simulink model "sgMdl_IO750_EtherCATDriveControl"  (R2024b)
settings: Solver=FixedStepAuto  StartTime=0.0  StopTime=inf  RelTol=1e-3  EnableMultiTasking=on
undefined symbols (not defined in the file): AUS0, AUS1, C, DiscIntNeverNeededParam, padding, sigbuilder_block, Statuswort, Steuerwort, Ts
libraries: slrealtimeethercatlib x13, simulink x10, speedgoatlib_IO750 x5, speedgoatlib_shared x1
Description:
  | IO750 - EtherCAT Drive Control
settings Model: ModifiedByFormat=Speedgoat  SimulationMode=external  Creator=Speedgoat  LastModifiedBy=Speedgoat
settings SolverCC: ConcurrentTasks=on  AlgebraicLoopSolver=TrustRegion  PositivePriorityOrder=on  AutoInsertRateTranBlk=on
settings DataIOCC: SaveFormat=StructureWithTime
settings OptimizationCC: BlockReduction=off  OptimizeBlockIOStorage=off  BufferReuse=off  GlobalBufferReuse=off  ExpressionFolding=off  LocalBlockOutputs=off  OptimizeDataStoreBuffers=off  BusAssignmentInplaceUpdate=off
settings DebuggingCC: TasksWithSamePriorityMsg=none  UnconnectedInputMsg=warning  UnconnectedOutputMsg=warning  UnconnectedLineMsg=warning
settings HardwareCC: ProdBitPerLong=64  ProdLongLongMode=on  ProdHWDeviceType=Intel->x86-64 (Linux 64)
settings ModelReferenceCC: EnableRefExpFcnMdlSchedulingChecks=on
settings RTWCC: Description=Speedgoat Real-Time Target Machine  SystemTargetFile=speedgoat.tlc  TemplateMakefile=slrealtime_default_tmf  Toolchain=Simulink Real-Time Toolchain  BuildConfiguration=Faster Runs  TargetLang=C++  GPUComputeCapability=3.5  DLArmComputeVersion=19.05
settings SimulinkRealTimeTargetCC: SubcomponentCodeInterfacePackaging=Reusable function  InstructionSetFMA=off  LogToMDFFile=off  SLRTFileLogMaxRuns=10  UseGCCFastMath=on
settings ConfigComp: CovBoundaryAbsTol=1.0e-5

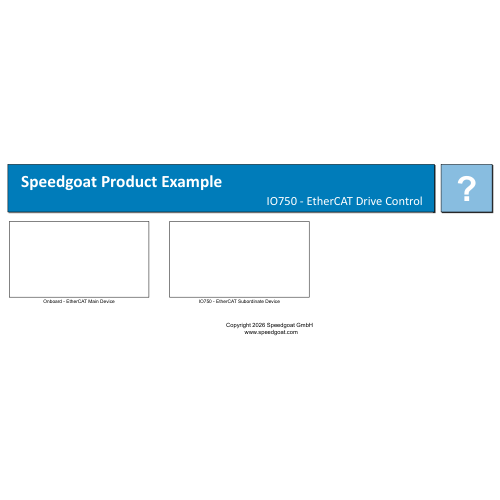
[thumbnail: Simulink's stored preview of the top-level diagram]
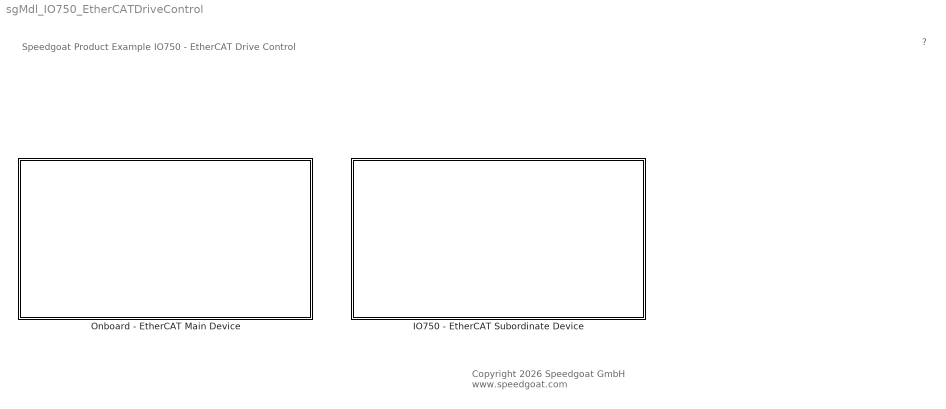
== system sgMdl_IO750_EtherCATDriveControl ==
  note: Speedgoat Product Example
      | IO750 - EtherCAT Drive Control
  note: ?
  note: Copyright 2026 Speedgoat GmbH
      |  www.speedgoat.com
  IO750 - EtherCAT Subordinate Device : Subsystem
  Onboard - EtherCAT Main Device : Subsystem

== system sgMdl_IO750_EtherCATDriveControl/IO750 - EtherCAT Subordinate Device ==
  Communication : Subsystem
  Controlled System : Subsystem
  wires:
  Communication/1(CommandValues) -> Controlled System/1(CommandValues)
  Controlled System/1(ActualValues) -> Communication/1(ActualValues)

== system sgMdl_IO750_EtherCATDriveControl/Onboard - EtherCAT Main Device ==
  Communication : Subsystem
  Controller : Subsystem
  wires:
  Communication/1(ActualValues) -> Controller/1(ActualValues)
  Controller/1(CommandValues) -> Communication/1(CommandValues)
  Communication/2(Status) -> Controller/2(Status)

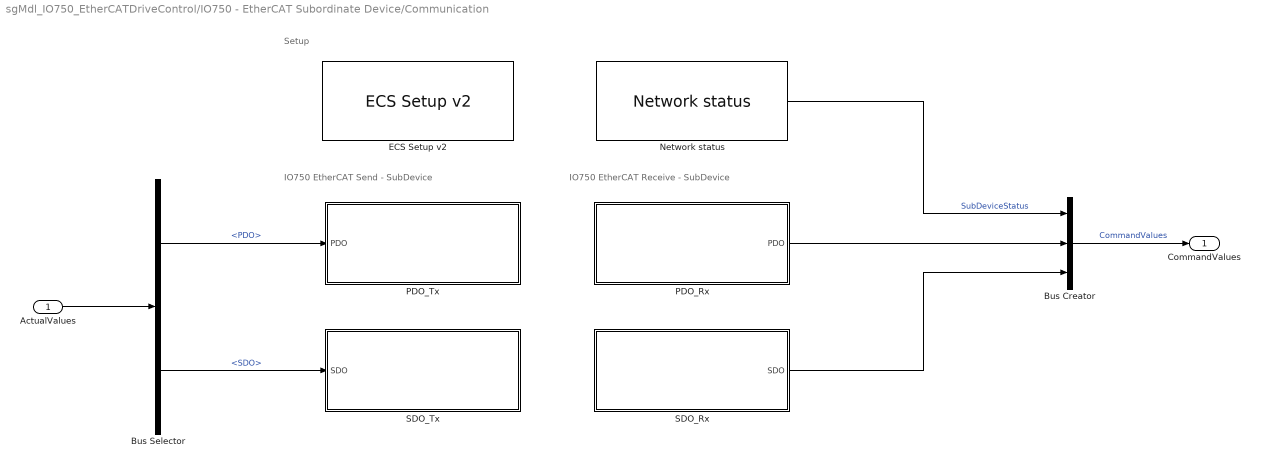
== system sgMdl_IO750_EtherCATDriveControl/IO750 - EtherCAT Subordinate Device/Communication ==
  note: IO750 EtherCAT Receive - SubDevice
  note: IO750 EtherCAT Send - SubDevice
  note: Setup
  ActualValues : Inport
  Bus Creator : BusCreator  Inputs=3
  Bus Selector : BusSelector  OutputSignals=PDO,SDO
  "ECS Setup v2 " : speedgoatlib_IO750/ECS Setup v2   id=1  drvLetter=C:  configurationMode=Warmstart  busSlot=-1  busStartup=Automatic  dcSync=off  RxSync=Free run  TxSync=Free run  vendorName='Speedgoat'  groupName='Automation'  typeName='Drive'  vendorID=hex2dec('11111111')  productCode=hex2dec('22222222')  revisionNo=hex2dec('33333333')  serialNo=102030405  stationAlias=0  deviceIdent=0  rxPdoMapping={ 'rxServo', 'ControlWord', 'uint16'; 'rxServo', 'ControlSpeed', 'double'; 'rxUtil', 'Alive', 'uint32' }  rxPdoCfg=0  rxPdoNames=,Steuerwort,Steuerwort,Statuswort  rxVarNames=,AUS0,padding,AUS1  txPdoMapping={ 'txServo', 'StatusWord', 'uint16'; 'txServo', 'ActualSpeed', 'double'; 'txServo', 'Position', 'int32'; 'txUtil', 'Alive', 'uint32' }  txPdoCfg=0  txPdoNames=0  txVarNames=0  sdoMapping={ '4000', '00', 'Servo', 'double', '1', 'read-write', 'none'; '4000', '02', 'Mode', 'uint8', '0', 'read-write', 'read'; '4000', '03', 'Homing', 'boolean', '0', 'read-write', 'read'; '4005', '00', 'Serial Number', 'uint32', '102030405', 'read', 'write' }  sdoCfg=0  sdoNames=0  qtyMods=[1,0,0]  moduleType=IO750  protocol=IO750  firmware=EtherCAT Slave
      settings: SourceProductName=Simulink Real-Time: Speedgoat I/O Blockset
  Network status : speedgoatlib_shared/IO75X/Network status  id=1  get_status=on  set_status=off  timeout=0.01  ts=Ts
  PDO_Rx : Subsystem
  PDO_Tx : Subsystem
  SDO_Rx : Subsystem
  SDO_Tx : Subsystem
  CommandValues : Outport
  wires:
  Bus Creator/1 -> CommandValues/1  "CommandValues"
  Bus Selector/1 -> PDO_Tx/1(PDO)  "<PDO>"
  Bus Selector/2 -> SDO_Tx/1(SDO)  "<SDO>"
  ActualValues/1 -> Bus Selector/1
  PDO_Rx/1(PDO) -> Bus Creator/2
  SDO_Rx/1(SDO) -> Bus Creator/3
  Network status/1 -> Bus Creator/1  "SubDeviceStatus"

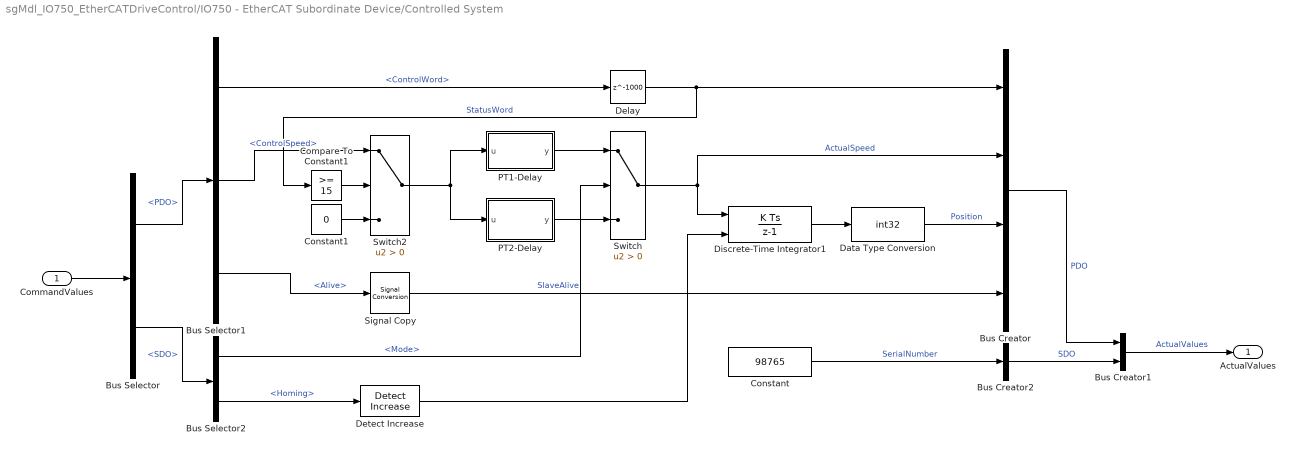
== system sgMdl_IO750_EtherCATDriveControl/IO750 - EtherCAT Subordinate Device/Controlled System ==
  CommandValues : Inport
  Bus Creator : BusCreator  Inputs=4
  Bus Creator1 : BusCreator  Inputs=2
  Bus Creator2 : BusCreator  Inputs=1
  Bus Selector : BusSelector  OutputSignals=PDO,SDO
  Bus Selector1 : BusSelector  OutputSignals=ControlWord,ControlSpeed,Alive
  Bus Selector2 : BusSelector  OutputSignals=Mode,Homing
  Compare To Constant1 : simulink/Logic and Bit Operations/Compare To Constant  relop=>=  const=15  OutDataTypeStr=boolean
  Constant : Constant  Value=98765  OutDataTypeStr=uint32  SampleTime=Ts
  Constant1 : Constant  Value=0
  Data Type Conversion : DataTypeConversion  OutDataTypeStr=int32  SaturateOnIntegerOverflow=off  RndMeth=Floor
  Delay : Delay  DelayLength=1000
  Detect Increase : simulink/Logic and Bit Operations/Detect Increase  vinit=0.0  OutDataTypeStr=boolean
  Discrete-Time Integrator1 : DiscreteIntegrator  ExternalReset=rising  SampleTime=-1  ICPrevOutput=DiscIntNeverNeededParam  ICPrevScaledInput=DiscIntNeverNeededParam
  PT1-Delay : Subsystem
  PT2-Delay : Subsystem
  Signal Copy : SignalConversion  OverrideOpt=off
  Switch : Switch  Criteria=u2 > Threshold  SaturateOnIntegerOverflow=off  InputSameDT=off
  Switch2 : Switch  Criteria=u2 > Threshold  SaturateOnIntegerOverflow=off  InputSameDT=off
  ActualValues : Outport
  wires:
  Bus Selector1/3 -> Signal Copy/1  "<Alive>"
  Signal Copy/1 -> Bus Creator/4  "SlaveAlive"
  Constant/1 -> Bus Creator2/1  "SerialNumber"
  Switch/1 -> Discrete-Time Integrator1/1, Bus Creator/2  "ActualSpeed"
  CommandValues/1 -> Bus Selector/1
  Bus Selector/1 -> Bus Selector1/1  "<PDO>"
  Bus Selector/2 -> Bus Selector2/1  "<SDO>"
  Bus Creator/1 -> Bus Creator1/1  "PDO"
  Bus Creator2/1 -> Bus Creator1/2  "SDO"
  Bus Creator1/1 -> ActualValues/1  "ActualValues"
  Bus Selector2/2 -> Detect Increase/1  "<Homing>"
  Bus Selector1/1 -> Delay/1  "<ControlWord>"
  Discrete-Time Integrator1/1 -> Data Type Conversion/1
  PT1-Delay/1(y) -> Switch/1
  PT2-Delay/1(y) -> Switch/3
  Bus Selector2/1 -> Switch/2  "<Mode>"
  Detect Increase/1 -> Discrete-Time Integrator1/2
  Delay/1 -> Compare To Constant1/1, Bus Creator/1  "StatusWord"
  Data Type Conversion/1 -> Bus Creator/3  "Position"
  Switch2/1 -> PT2-Delay/1(u), PT1-Delay/1(u)
  Compare To Constant1/1 -> Switch2/2
  Bus Selector1/2 -> Switch2/1  "<ControlSpeed>"
  Constant1/1 -> Switch2/3

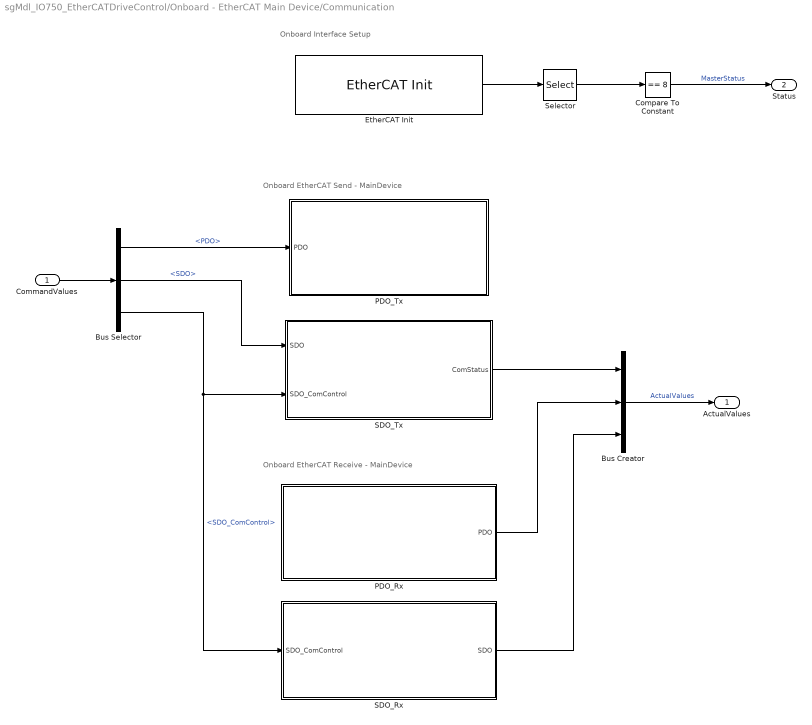
== system sgMdl_IO750_EtherCATDriveControl/Onboard - EtherCAT Main Device/Communication ==
  note: Onboard Interface Setup
  note: Onboard EtherCAT Send - MainDevice
  note: Onboard EtherCAT Receive - MainDevice
  CommandValues : Inport
  Bus Creator : BusCreator  Inputs=3
  Bus Selector : BusSelector  OutputSignals=PDO,SDO,SDO_ComControl
  Compare To Constant : simulink/Logic and Bit Operations/Compare To Constant  relop===  const=8  OutDataTypeStr=boolean
  "EtherCAT Init " : slrealtimeethercatlib/EtherCAT Init  Priority=0  config_file=IO750_EtherCATDriveControl_eni.xml  device_id=0  portnum=1  initstate=2  dctuning=0  enaDebug=0  logFile='c:\dbglog.txt'  sample_time=0.010000  DCMode=0
  PDO_Rx : Subsystem
  PDO_Tx : Subsystem
  SDO_Rx : Subsystem
  SDO_Tx : Subsystem
  Selector : Selector  InputPortWidth=6  IndexOptions=Index vector (dialog)  Indices=2  OutputSizes=1
  ActualValues : Outport
  Status : Outport  Port=2
  wires:
  Bus Creator/1 -> ActualValues/1  "ActualValues"
  CommandValues/1 -> Bus Selector/1
  Bus Selector/1 -> PDO_Tx/1(PDO)  "<PDO>"
  Bus Selector/2 -> SDO_Tx/1(SDO)  "<SDO>"
  Bus Selector/3 -> SDO_Rx/1(SDO_ComControl), SDO_Tx/2(SDO_ComControl)  "<SDO_ComControl>"
  PDO_Rx/1(PDO) -> Bus Creator/2
  SDO_Tx/1(ComStatus) -> Bus Creator/1
  SDO_Rx/1(SDO) -> Bus Creator/3
  "EtherCAT Init "/1 -> Selector/1
  Selector/1 -> Compare To Constant/1
  Compare To Constant/1 -> Status/1  "MasterStatus"

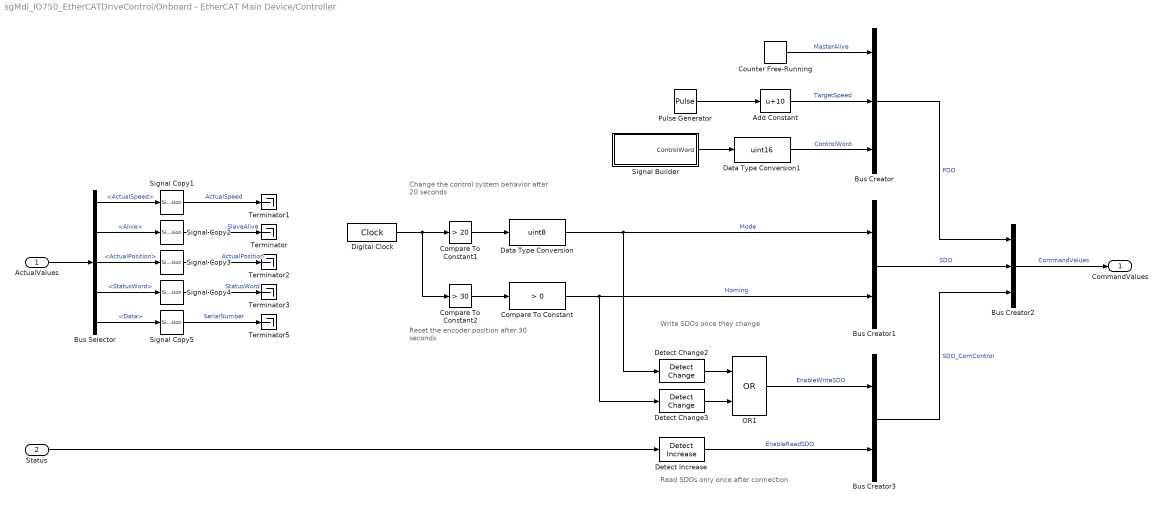
== system sgMdl_IO750_EtherCATDriveControl/Onboard - EtherCAT Main Device/Controller ==
  note: Change the control system behavior after 20 seconds
  note: Reset the encoder position after 30 seconds
  note: Read SDOs only once after connection
  note: Write SDOs once they change
  ActualValues : Inport
  Status : Inport  Port=2
  Add Constant : Bias  Bias=10  SaturateOnIntegerOverflow=off
  Bus Creator : BusCreator  Inputs=3
  Bus Creator1 : BusCreator  Inputs=2
  Bus Creator2 : BusCreator  Inputs=3
  Bus Creator3 : BusCreator  Inputs=2
  Bus Selector : BusSelector  OutputSignals=PDO.ActualSpeed,PDO.Alive,PDO.ActualPosition,PDO.StatusWord,SDO.Serial_Number.Data
  Compare To Constant : simulink/Logic and Bit Operations/Compare To Constant  relop=>  const=0  OutDataTypeStr=boolean
  Compare To Constant1 : simulink/Logic and Bit Operations/Compare To Constant  relop=>  const=20  OutDataTypeStr=boolean
  Compare To Constant2 : simulink/Logic and Bit Operations/Compare To Constant  relop=>  const=30  OutDataTypeStr=boolean
  Counter Free-Running : simulink/Sources/Counter Free-Running  NumBits=32  tsamp=Ts
  Data Type Conversion : DataTypeConversion  OutDataTypeStr=uint8  SaturateOnIntegerOverflow=off  RndMeth=Floor
  Data Type Conversion1 : DataTypeConversion  OutDataTypeStr=uint16  SaturateOnIntegerOverflow=off  RndMeth=Floor
  Detect Change2 : simulink/Logic and Bit Operations/Detect Change  vinit=0  OutDataTypeStr=boolean
  Detect Change3 : simulink/Logic and Bit Operations/Detect Change  vinit=0  OutDataTypeStr=boolean
  Detect Increase : simulink/Logic and Bit Operations/Detect Increase  vinit=0.0  OutDataTypeStr=boolean
  Digital Clock : DigitalClock  SampleTime=Ts
  OR1 : Logic  Operator=OR  IconShape=distinctive  AllPortsSameDT=off  OutDataTypeStr=boolean
  Pulse Generator : DiscretePulseGenerator  Amplitude=40  Period=5*1/Ts  PulseWidth=3*1/Ts  SampleTime=Ts
  Signal Builder : Subsystem  Tag=STV Subsys  LoadFcn=sigbuilder_block('load');  StartFcn=sigbuilder_block('start');  StopFcn=sigbuilder_block('stop');  ClipboardFcn=sigbuilder_block('clipboard');  mask(Sigbuilder block){tuvar=[0:10]}
      mask help: Simulink:masks:SigbuilderBlock_MD
      mask init:
      | if ~strcmp(get_param(bdroot(gcbh),'SimulationStatus'),'stopped') tuvar = sigbuilder_block('maskInit'); end
      settings: CopyFcn=sigbuilder_block('copy');  DeleteFcn=sigbuilder_block('delete');  ModelCloseFcn=sigbuilder_block('modelClose');  PreSaveFcn=sigbuilder_block('preSave');  PauseFcn=sigbuilder_block('pause');  ContinueFcn=sigbuilder_block('continue');  NameChangeFcn=sigbuilder_block('namechange');  OpenFcn=sigbuilder_block('open',[6 30 1428 681.75 ]);  CloseFcn=sigbuilder_block('close');
      mask Display: plot(0, 0, 100, 100,[2, 2, 32, 32, 2], [68, 8, 8, 68, 68],[32, 2], [38, 38], [32, 19, 2],[53, 60, 44], [32, 17, 17, 2],[16, 16, 31, 31]);txt = getActiveGroup(gcbh);text(2, 100, txt,'verticalAlignment', 'top');
  Signal Copy{1..5} (5 alike) : SignalConversion  OverrideOpt=off
  Terminator{,1..3,5} (5 alike) : Terminator
  CommandValues : Outport
  wires:
  Signal Builder/1(ControlWord) -> Data Type Conversion1/1
  Counter Free-Running/1 -> Bus Creator/1  "MasterAlive"
  Bus Creator/1 -> Bus Creator2/1  "PDO"
  Compare To Constant1/1 -> Data Type Conversion/1
  Compare To Constant2/1 -> Compare To Constant/1
  Bus Creator1/1 -> Bus Creator2/2  "SDO"
  Bus Creator2/1 -> CommandValues/1  "CommandValues"
  OR1/1 -> Bus Creator3/1  "EnableWriteSDO"
  Detect Increase/1 -> Bus Creator3/2  "EnableReadSDO"
  Bus Creator3/1 -> Bus Creator2/3  "SDO_ComControl"
  ActualValues/1 -> Bus Selector/1
  Bus Selector/2 -> Signal Copy2/1  "<Alive>"
  Bus Selector/1 -> Signal Copy1/1  "<ActualSpeed>"
  Bus Selector/3 -> Signal Copy3/1  "<ActualPosition>"
  Bus Selector/4 -> Signal Copy4/1  "<StatusWord>"
  Bus Selector/5 -> Signal Copy5/1  "<Data>"
  Signal Copy1/1 -> Terminator1/1  "ActualSpeed"
  Signal Copy3/1 -> Terminator2/1  "ActualPosition"
  Signal Copy4/1 -> Terminator3/1  "StatusWord"
  Signal Copy5/1 -> Terminator5/1  "SerialNumber"
  Signal Copy2/1 -> Terminator/1  "SlaveAlive"
  Add Constant/1 -> Bus Creator/2  "TargetSpeed"
  Status/1 -> Detect Increase/1
  Data Type Conversion/1 -> Bus Creator1/1, Detect Change2/1  "Mode"
  Compare To Constant/1 -> Bus Creator1/2, Detect Change3/1  "Homing"
  Detect Change2/1 -> OR1/1
  Detect Change3/1 -> OR1/2
  Pulse Generator/1 -> Add Constant/1
  Digital Clock/1 -> Compare To Constant2/1, Compare To Constant1/1
  Data Type Conversion1/1 -> Bus Creator/3  "ControlWord"

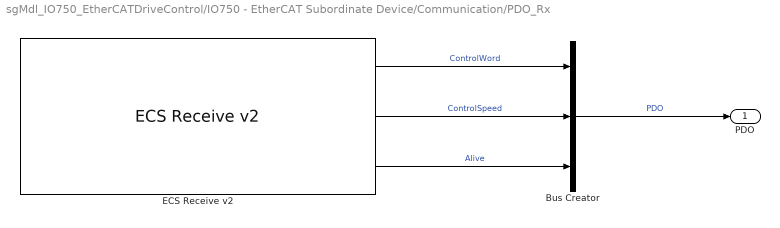
== system sgMdl_IO750_EtherCATDriveControl/IO750 - EtherCAT Subordinate Device/Communication/PDO_Rx ==
  Bus Creator : BusCreator  Inputs=3
  "ECS Receive v2 " : speedgoatlib_IO750/ECS Receive v2   id=1  portType=Separate signals  sampleTime=Ts  pdoTable={ 'rxServo', 'ControlWord', 'uint16'; 'rxServo', 'ControlSpeed', 'double'; 'rxUtil', 'Alive', 'uint32' }
      settings: SourceProductName=Simulink Real-Time: Speedgoat I/O Blockset
  PDO : Outport
  wires:
  "ECS Receive v2 "/1 -> Bus Creator/1  "ControlWord"
  "ECS Receive v2 "/3 -> Bus Creator/3  "Alive"
  Bus Creator/1 -> PDO/1  "PDO"
  "ECS Receive v2 "/2 -> Bus Creator/2  "ControlSpeed"

== system sgMdl_IO750_EtherCATDriveControl/IO750 - EtherCAT Subordinate Device/Communication/PDO_Tx ==
  PDO : Inport
  Bus Selector1 : BusSelector  OutputSignals=StatusWord,ActualSpeed,Position,SlaveAlive
  "ECS Send v2 " : speedgoatlib_IO750/ECS Send v2   id=1  portType=Separate signals  sampleTime=-1  pdoTable={ 'txServo', 'StatusWord', 'uint16'; 'txServo', 'ActualSpeed', 'double'; 'txServo', 'Position', 'int32'; 'txUtil', 'Alive', 'uint32' }
      settings: SourceProductName=Simulink Real-Time: Speedgoat I/O Blockset
  wires:
  PDO/1 -> Bus Selector1/1
  Bus Selector1/4 -> "ECS Send v2 "/4  "<SlaveAlive>"
  Bus Selector1/1 -> "ECS Send v2 "/1  "<StatusWord>"
  Bus Selector1/3 -> "ECS Send v2 "/3  "<Position>"
  Bus Selector1/2 -> "ECS Send v2 "/2  "<ActualSpeed>"

== system sgMdl_IO750_EtherCATDriveControl/IO750 - EtherCAT Subordinate Device/Communication/SDO_Rx ==
  Bus Creator : BusCreator  Inputs=2
  "ECS Read SDO " : speedgoatlib_IO750/ECS Read SDO   id=1  sampleTime=Ts  sdoTable={ '4000', '00', 'Servo', 'double', '1', 'read-write', 'none'; '4000', '02', 'Mode', 'uint8', '0', 'read-write', 'read'; '4000', '03', 'Homing', 'boolean', '0', 'read-write', 'read'; '4005', '00', 'Serial Number', 'uint32', '102030405', 'read', 'write' }  sdoCfg=0
      settings: SourceProductName=Simulink Real-Time: Speedgoat I/O Blockset
  SDO : Outport
  wires:
  "ECS Read SDO "/2 -> Bus Creator/2  "Homing"
  Bus Creator/1 -> SDO/1  "SDO"
  "ECS Read SDO "/1 -> Bus Creator/1  "Mode"

== system sgMdl_IO750_EtherCATDriveControl/IO750 - EtherCAT Subordinate Device/Communication/SDO_Tx ==
  SDO : Inport
  Bus Selector2 : BusSelector  OutputSignals=SerialNumber
  "ECS Write SDO " : speedgoatlib_IO750/ECS Write SDO   id=1  sampleTime=-1  sdoTable={ '4000', '00', 'Servo', 'double', '1', 'read-write', 'none'; '4000', '02', 'Mode', 'uint8', '0', 'read-write', 'read'; '4000', '03', 'Homing', 'boolean', '0', 'read-write', 'read'; '4005', '00', 'Serial Number', 'uint32', '102030405', 'read', 'write' }  sdoCfg=0
      settings: SourceProductName=Simulink Real-Time: Speedgoat I/O Blockset
  wires:
  Bus Selector2/1 -> "ECS Write SDO "/1  "<SerialNumber>"
  SDO/1 -> Bus Selector2/1

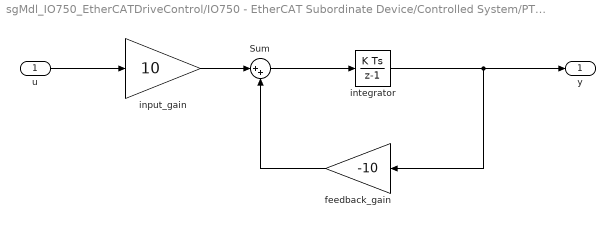
== system sgMdl_IO750_EtherCATDriveControl/IO750 - EtherCAT Subordinate Device/Controlled System/PT1-Delay ==
  u : Inport
  Sum : Sum  Inputs=|++
  "feedback_gain " : Gain  Gain=-10
  input_gain : Gain  Gain=10
  integrator : DiscreteIntegrator  SampleTime=0.001  ICPrevOutput=DiscIntNeverNeededParam  ICPrevScaledInput=DiscIntNeverNeededParam
  y : Outport  VectorParamsAs1DForOutWhenUnconnected=off
  wires:
  u/1 -> input_gain/1
  "feedback_gain "/1 -> Sum/2
  integrator/1 -> "feedback_gain "/1, y/1
  Sum/1 -> integrator/1
  input_gain/1 -> Sum/1

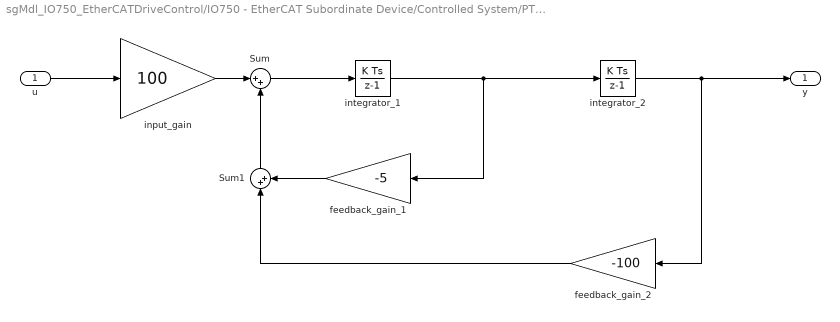
== system sgMdl_IO750_EtherCATDriveControl/IO750 - EtherCAT Subordinate Device/Controlled System/PT2-Delay ==
  u : Inport
  Sum : Sum  Inputs=|++
  Sum1 : Sum  Inputs=|++
  feedback_gain_1 : Gain  Gain=-5
  feedback_gain_2 : Gain  Gain=-100
  input_gain : Gain  Gain=100
  integrator_1 : DiscreteIntegrator  gainval=2  SampleTime=0.001  ICPrevOutput=DiscIntNeverNeededParam  ICPrevScaledInput=DiscIntNeverNeededParam
  integrator_2 : DiscreteIntegrator  gainval=2  SampleTime=0.001  ICPrevOutput=DiscIntNeverNeededParam  ICPrevScaledInput=DiscIntNeverNeededParam
  y : Outport  VectorParamsAs1DForOutWhenUnconnected=off
  wires:
  feedback_gain_2/1 -> Sum1/1
  integrator_2/1 -> y/1, feedback_gain_2/1
  feedback_gain_1/1 -> Sum1/2
  input_gain/1 -> Sum/1
  Sum/1 -> integrator_1/1
  integrator_1/1 -> integrator_2/1, feedback_gain_1/1
  Sum1/1 -> Sum/2
  u/1 -> input_gain/1

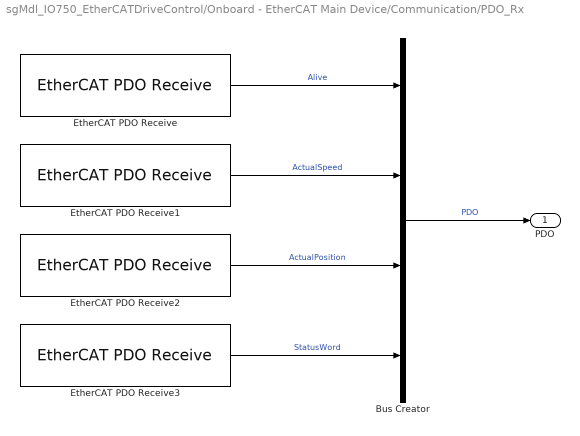
== system sgMdl_IO750_EtherCATDriveControl/Onboard - EtherCAT Main Device/Communication/PDO_Rx ==
  Bus Creator : BusCreator  Inputs=4
  EtherCAT PDO Receive : slrealtimeethercatlib/EtherCAT PDO Receive  Priority=2  sig_name=Box 1 (Drive).txUtil.Alive  sig_offset=632  sig_type=uint32  type_size=32  sig_dim=1  device_id=0  sample_time=0.001000
  EtherCAT PDO Receive1 : slrealtimeethercatlib/EtherCAT PDO Receive  Priority=2  sig_name=Box 1 (Drive).txServo.ActualSpeed  sig_offset=536  sig_type=double  type_size=64  sig_dim=1  device_id=0  sample_time=0.001000
  EtherCAT PDO Receive2 : slrealtimeethercatlib/EtherCAT PDO Receive  Priority=2  sig_name=Box 1 (Drive).txServo.Position  sig_offset=600  sig_type=int32  type_size=32  sig_dim=1  device_id=0  sample_time=0.001000
  EtherCAT PDO Receive3 : slrealtimeethercatlib/EtherCAT PDO Receive  Priority=2  sig_name=Box 1 (Drive).txServo.StatusWord  sig_offset=520  sig_type=uint16  type_size=16  sig_dim=1  device_id=0  sample_time=0.001000
  PDO : Outport
  wires:
  EtherCAT PDO Receive/1 -> Bus Creator/1  "Alive"
  EtherCAT PDO Receive2/1 -> Bus Creator/3  "ActualPosition"
  EtherCAT PDO Receive1/1 -> Bus Creator/2  "ActualSpeed"
  Bus Creator/1 -> PDO/1  "PDO"
  EtherCAT PDO Receive3/1 -> Bus Creator/4  "StatusWord"

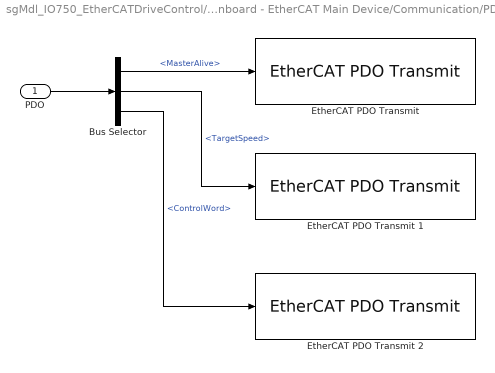
== system sgMdl_IO750_EtherCATDriveControl/Onboard - EtherCAT Main Device/Communication/PDO_Tx ==
  PDO : Inport
  Bus Selector : BusSelector  OutputSignals=MasterAlive,TargetSpeed,ControlWord
  "EtherCAT PDO Transmit " : slrealtimeethercatlib/EtherCAT PDO Transmit  Priority=3  sig_name=Box 1 (Drive).rxUtil.Alive  sig_offset=392  sig_type=uint32  type_size=32  sig_dim=1  device_id=0  sample_time=0.001
  EtherCAT PDO Transmit 1 : slrealtimeethercatlib/EtherCAT PDO Transmit  Priority=3  sig_name=Box 1 (Drive).rxServo.ControlSpeed  sig_offset=328  sig_type=double  type_size=64  sig_dim=1  device_id=0  sample_time=0.001000
  EtherCAT PDO Transmit 2 : slrealtimeethercatlib/EtherCAT PDO Transmit  Priority=3  sig_name=Box 1 (Drive).rxServo.ControlWord  sig_offset=312  sig_type=uint16  type_size=16  sig_dim=1  device_id=0  sample_time=0.001000
  wires:
  PDO/1 -> Bus Selector/1
  Bus Selector/2 -> EtherCAT PDO Transmit 1/1  "<TargetSpeed>"
  Bus Selector/1 -> "EtherCAT PDO Transmit "/1  "<MasterAlive>"
  Bus Selector/3 -> EtherCAT PDO Transmit 2/1  "<ControlWord>"

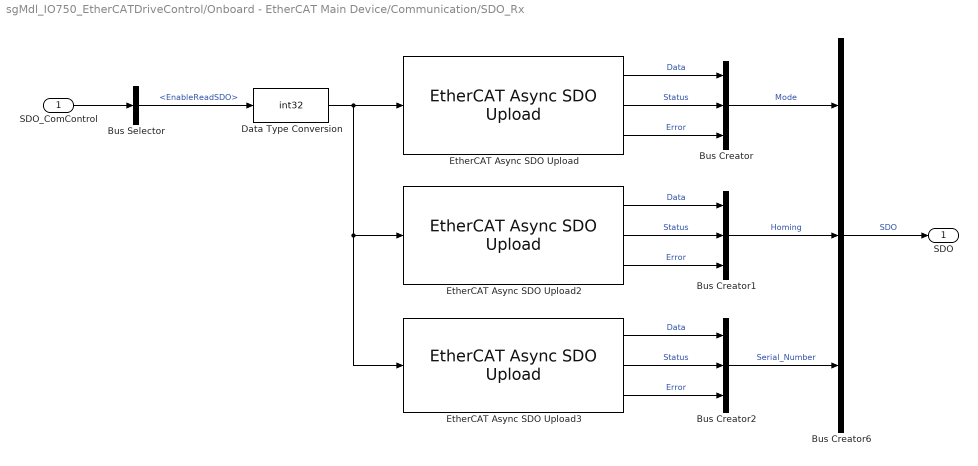
== system sgMdl_IO750_EtherCATDriveControl/Onboard - EtherCAT Main Device/Communication/SDO_Rx ==
  SDO_ComControl : Inport
  Bus Creator{,1..2,6} (4 alike) : BusCreator  Inputs=3
  Bus Selector : BusSelector  OutputSignals=EnableReadSDO
  Data Type Conversion : DataTypeConversion  OutDataTypeStr=int32  SaturateOnIntegerOverflow=off  RndMeth=Floor
  EtherCAT Async SDO Upload : slrealtimeethercatlib/EtherCAT Async SDO Upload  index=hex2dec('4000')  subIndex=hex2dec('2')  sig_type=uint8  sig_dim=1  device_id=0  subdevice_name=Box 1 (Drive)  sample_time=-1  subdevice_addr=1001  selected_subdevice=Term 1 (EK1100)  timeout=5000  subdevice_found=1  complete=0
  EtherCAT Async SDO Upload2 : slrealtimeethercatlib/EtherCAT Async SDO Upload  index=hex2dec('4000')  subIndex=hex2dec('03')  sig_type=boolean  sig_dim=1  device_id=0  subdevice_name=Box 1 (Drive)  sample_time=-1  subdevice_addr=1001  selected_subdevice=Term 1 (EK1100)  timeout=5000  subdevice_found=1  complete=0
  EtherCAT Async SDO Upload3 : slrealtimeethercatlib/EtherCAT Async SDO Upload  index=hex2dec('4005')  subIndex=hex2dec('00')  sig_type=uint32  sig_dim=1  device_id=0  subdevice_name=Box 1 (Drive)  sample_time=-1  subdevice_addr=1001  selected_subdevice=Term 1 (EK1100)  timeout=5000  subdevice_found=1  complete=0
  SDO : Outport
  wires:
  Bus Selector/1 -> Data Type Conversion/1  "<EnableReadSDO>"
  EtherCAT Async SDO Upload/1 -> Bus Creator/1  "Data"
  Bus Creator/1 -> Bus Creator6/1  "Mode"
  Bus Creator6/1 -> SDO/1  "SDO"
  Bus Creator1/1 -> Bus Creator6/2  "Homing"
  EtherCAT Async SDO Upload2/2 -> Bus Creator1/2  "Status"
  Bus Creator2/1 -> Bus Creator6/3  "Serial_Number"
  EtherCAT Async SDO Upload2/1 -> Bus Creator1/1  "Data"
  EtherCAT Async SDO Upload/3 -> Bus Creator/3  "Error"
  EtherCAT Async SDO Upload/2 -> Bus Creator/2  "Status"
  EtherCAT Async SDO Upload3/2 -> Bus Creator2/2  "Status"
  EtherCAT Async SDO Upload3/1 -> Bus Creator2/1  "Data"
  EtherCAT Async SDO Upload3/3 -> Bus Creator2/3  "Error"
  EtherCAT Async SDO Upload2/3 -> Bus Creator1/3  "Error"
  SDO_ComControl/1 -> Bus Selector/1
  Data Type Conversion/1 -> EtherCAT Async SDO Upload3/1, EtherCAT Async SDO Upload2/1, EtherCAT Async SDO Upload/1

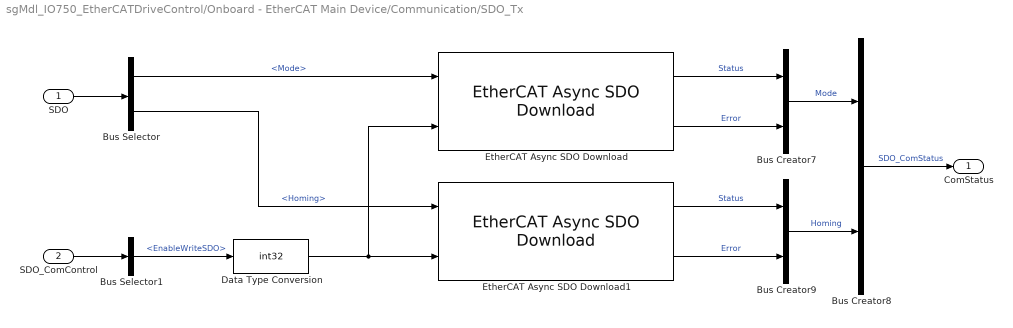
== system sgMdl_IO750_EtherCATDriveControl/Onboard - EtherCAT Main Device/Communication/SDO_Tx ==
  SDO : Inport
  SDO_ComControl : Inport  Port=2
  Bus Creator7 : BusCreator  Inputs=2
  Bus Creator8 : BusCreator  Inputs=2
  Bus Creator9 : BusCreator  Inputs=2
  Bus Selector : BusSelector  OutputSignals=Mode,Homing
  Bus Selector1 : BusSelector  OutputSignals=EnableWriteSDO
  Data Type Conversion : DataTypeConversion  OutDataTypeStr=int32  SaturateOnIntegerOverflow=off  RndMeth=Floor
  EtherCAT Async SDO Download : slrealtimeethercatlib/EtherCAT Async SDO Download  index=hex2dec('4000')  subIndex=hex2dec('2')  sig_type=uint8  sig_dim=1  device_id=0  subdevice_name=Box 1 (Drive)  sample_time=-1  subdevice_addr=1001  selected_subdevice=Term 1 (EK1100)  timeout=5000  subdevice_found=1  complete=0
  EtherCAT Async SDO Download1 : slrealtimeethercatlib/EtherCAT Async SDO Download  index=hex2dec('4000')  subIndex=hex2dec('4003')  sig_type=boolean  sig_dim=1  device_id=0  subdevice_name=Box 1 (Drive)  sample_time=-1  subdevice_addr=1001  selected_subdevice=Term 1 (EK1100)  timeout=5000  subdevice_found=1  complete=0
  ComStatus : Outport
  wires:
  EtherCAT Async SDO Download/2 -> Bus Creator7/2  "Error"
  Bus Creator9/1 -> Bus Creator8/2  "Homing"
  Bus Creator7/1 -> Bus Creator8/1  "Mode"
  EtherCAT Async SDO Download/1 -> Bus Creator7/1  "Status"
  EtherCAT Async SDO Download1/2 -> Bus Creator9/2  "Error"
  EtherCAT Async SDO Download1/1 -> Bus Creator9/1  "Status"
  Bus Selector/1 -> EtherCAT Async SDO Download/1  "<Mode>"
  Bus Selector/2 -> EtherCAT Async SDO Download1/1  "<Homing>"
  Bus Selector1/1 -> Data Type Conversion/1  "<EnableWriteSDO>"
  Bus Creator8/1 -> ComStatus/1  "SDO_ComStatus"
  SDO/1 -> Bus Selector/1
  SDO_ComControl/1 -> Bus Selector1/1
  Data Type Conversion/1 -> EtherCAT Async SDO Download/2, EtherCAT Async SDO Download1/2

== system sgMdl_IO750_EtherCATDriveControl/Onboard - EtherCAT Main Device/Controller/Signal Builder ==
  Demux : Demux  Tag=STV Demux  Outputs=1
      settings: DisplayOption=none
  FromWs : FromWorkspace  Tag=STV FromWs  VariableName=tuvar
      SigBuilderData=|
      | common.afterFinalStr = 'Extrapolate'
      | common.sampleTime = 0
      | dataSet.timeRange = [0 10]
      | dataSet.name = 'Group 1'
      | sbobj.Groups.Name = 'Group 1'
      | sbobj.Groups.Signals.Name = 'ControlWord'
      | sbobj.Groups.Signals.XData = [0 1 1 3 3 5 5 7 7 10]
      | sbobj.Groups.Signals.YData = [0 0 2 2 3 3 7 7 15 15]
  ControlWord : Outport  Tag=STV Outport
  wires:
  Demux/1 -> ControlWord/1
  FromWs/1 -> Demux/1
